simulink model "experiment_toplevel"  (R2016a)
settings: Solver=ode15s  StartTime=0.0  StopTime=20  MaxStep=1e-2  RelTol=1e-4
PreLoadFcn:
  | minitaurParameters
values from neighbouring files (symbols this model uses):
  angular_ctrl_d = 1    [minitaurParameters.m]
  angular_ctrl_i = 1    [minitaurParameters.m]
  angular_ctrl_p = 100    [minitaurParameters.m]
  enc_zero_IA = -1.25*pi    (= -3.92699081699)    [minitaurParameters.m]
  enc_zero_IB = -0.25*pi    (= -0.785398163397)    [minitaurParameters.m]
  enc_zero_IIA = 1.25*pi    (= 3.92699081699)    [minitaurParameters.m]
  enc_zero_IIB = 1.25*pi    (= 3.92699081699)    [minitaurParameters.m]
  enc_zero_IIIA = 0.5*pi    (= 1.57079632679)    [minitaurParameters.m]
  enc_zero_IIIB = 1.5*pi    (= 4.71238898038)    [minitaurParameters.m]
  enc_zero_IVA = -0.25*pi    (= -0.785398163397)    [minitaurParameters.m]
  enc_zero_IVB = 0.5*pi    (= 1.57079632679)    [minitaurParameters.m]
  fore_lag = fore_lag_vals(j)    [experiment1.m]    (also in experiment1_parfor_accelerator.m = 0; minitaurParameters.m = 0.45)
  ground_frame_depth = 0.5    [minitaurParameters.m]
  ground_length = 100    [minitaurParameters.m]
  ground_width = 10    [minitaurParameters.m]
  init_theta_IA = -pi/4    (= -0.785398163397)    [minitaurParameters.m]
  init_theta_IB = pi/4    (= 0.785398163397)    [minitaurParameters.m]
  init_theta_IIA = -pi/4    (= -0.785398163397)    [minitaurParameters.m]
  init_theta_IIB = pi/4    (= 0.785398163397)    [minitaurParameters.m]
  init_theta_IIIA = -pi/4    (= -0.785398163397)    [minitaurParameters.m]
  init_theta_IIIB = pi/4    (= 0.785398163397)    [minitaurParameters.m]
  init_theta_IVA = -pi/4    (= -0.785398163397)    [minitaurParameters.m]
  init_theta_IVB = pi/4    (= 0.785398163397)    [minitaurParameters.m]
  l1 = 100e-3    (= 0.1)    [minitaurParameters.m]
  l2 = 200e-3    (= 0.2)    [minitaurParameters.m]
  leg_joint_radius = 3e-3    (= 0.003)    [minitaurParameters.m]
  lr_sync = 1    [experiment1.m]    (also in experiment1_parfor_accelerator.m; minitaurParameters.m = 0)
  model = 'experiment_toplevel'    [experiment1_parfor_accelerator.m]
  period = period_vals(i)    [experiment1.m]    (also in experiment1_parfor_accelerator.m = 1.5; minitaurParameters.m = 0.33)
  phi_0 = 0.5*asin(l1/l2)    [experiment1.m]    (also in experiment1_parfor_accelerator.m; minitaurParameters.m)
  r_0 = l2    [experiment1.m]    (also in experiment1_parfor_accelerator.m; minitaurParameters.m = 0.2)
  r_x = 0.3*l1    [experiment1.m]    (also in experiment1_parfor_accelerator.m = 0.5*l1; minitaurParameters.m = 0.05)
  r_y = 0.2*l1    [experiment1.m]    (also in experiment1_parfor_accelerator.m = 0.3*l1; minitaurParameters.m = 0.03)
  radial_ctrl_d = 1    [minitaurParameters.m]
  radial_ctrl_i = 1    [minitaurParameters.m]
  radial_ctrl_p = 80    [minitaurParameters.m]
  safety_limit = 10e-3    (= 0.01)    [minitaurParameters.m]
undefined symbols (not defined in the file or in its folder): Axis, Fn, minitaurParams, r_stance, r_swing, stance_frac, X, Y, Z
undefined symbols (not defined in the file): leg_joint_fric_bw, leg_joint_mu_k, leg_joint_mu_s, leg_joint_vel_thresh, motor_kt, motor_kv, motor_r, motor_torque_sat
libraries: sm_lib x453, fl_lib x132, nesl_utility x31, Contact_Forces_Lib x28, simulink x19
(part 2 of 13)

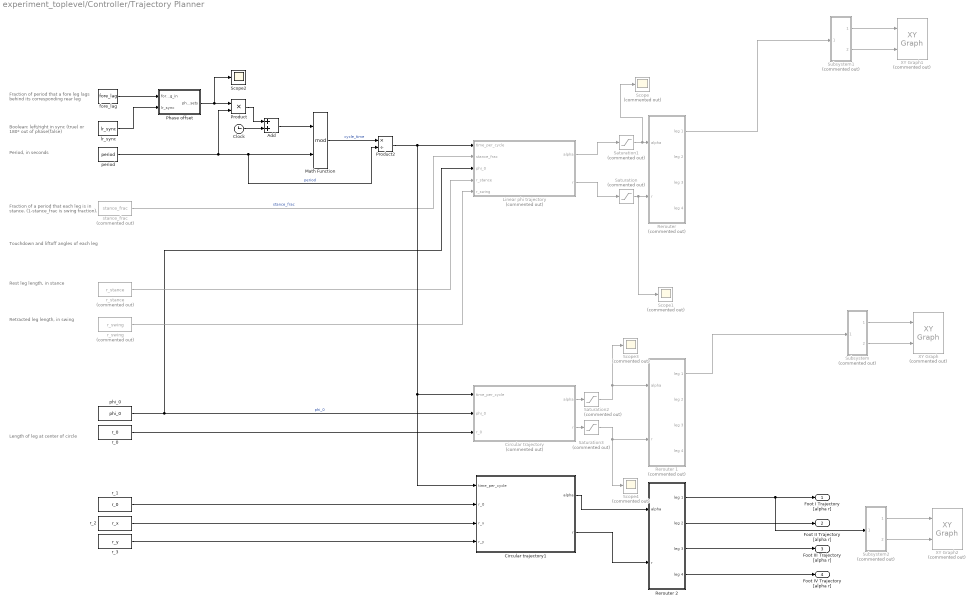
== system experiment_toplevel/Controller/Trajectory Planner ==
  note: Fraction of period that a fore leg
      | lags behind its corresponding rear leg
  note: Period, in seconds
  note: Fraction of a period that each leg is in stance. (1-stance_frac is swing fraction).
  note: Touchdown and liftoff angles of each leg
  note: Boolean: left/right in sync (true) or
      | 180* out of phase(false)
  note: Rest leg length, in stance
  note: Retracted leg length, in swing
  note: Length of leg at center of circle
  Add : Sum
  Circular trajectory : Subsystem  Commented=on
  Circular trajectory1 : Subsystem
  Clock : Clock
  Linear phi trajectory : Subsystem  Commented=on
  Math Function : Math  Operator=mod  SaturateOnIntegerOverflow=on
  Phase offset : Subsystem
  Product : Product
  Product2 : Product  Inputs=*/
  "Rerouter " : Subsystem  Commented=on
  Rerouter 1 : Subsystem  Commented=on
  Rerouter 2 : Subsystem
  Saturation : Saturate  Commented=on  UpperLimit=l2+l1  LowerLimit=l2-l1
  Saturation1 : Saturate  Commented=on  UpperLimit=3*pi/2  LowerLimit=pi/2
  Saturation2 : Saturate  Commented=on  UpperLimit=3*pi/2  LowerLimit=pi/2
  Saturation3 : Saturate  Commented=on  UpperLimit=l2+l1-safety_limit  LowerLimit=l2-l1+safety_limit
  Scope{,1,3..4} (4 alike) : Scope  Commented=on
  Scope2 : Scope
  Subsystem : Subsystem  Commented=on
  Subsystem1 : Subsystem  Commented=on
  Subsystem2 : Subsystem  Commented=on
  XY Graph : simulink/Sinks/XY Graph  Commented=on  xmin=-0.4  xmax=0.4  ymin=-0.5  ymax=0.1  st=-1
  XY Graph1 : simulink/Sinks/XY Graph  Commented=on  xmin=-0.4  xmax=0.4  ymin=-0.5  ymax=0.1  st=-1
  XY Graph2 : simulink/Sinks/XY Graph  Commented=on  xmin=-0.4  xmax=0.4  ymin=-0.5  ymax=0.1  st=-1
  fore_lag : Constant  Value=fore_lag
  lr_sync : Constant  Value=lr_sync  OutDataTypeStr=double
  period : Constant  Value=period  OutDataTypeStr=double
  phi_0 : Constant  Value=phi_0
  r_0 : Constant  Value=r_0
  r_1 : Constant  Value=r_0
  r_2 : Constant  Value=r_x
  r_3 : Constant  Value=r_y
  r_stance : Constant  Commented=on  Value=r_stance
  r_swing : Constant  Commented=on  Value=r_swing
  stance_frac : Constant  Commented=on  Value=stance_frac
  Foot I Trajectory [alpha r] : Outport
  Foot II Trajectory [alpha r] : Outport  Port=2
  Foot III Trajectory [alpha r] : Outport  Port=3
  Foot IV Trajectory [alpha r] : Outport  Port=4
  wires:
  period/1 -> Product/2, Product2/2, Math Function/2  "period"
  Clock/1 -> Add/2
  Add/1 -> Math Function/1
  Product/1 -> Add/1
  Phase offset/1(phase offsets) -> Scope2/1, Product/1
  lr_sync/1 -> Phase offset/2(lr_sync)
  Math Function/1 -> Product2/1  "cycle_time"
  stance_frac/1 -> Linear phi trajectory/2(stance_frac)  "stance_frac"
  phi_0/1 -> Linear phi trajectory/3(phi_0), Circular trajectory/2(phi_0)  "phi_0"
  r_stance/1 -> Linear phi trajectory/4("r_stance ")
  r_swing/1 -> Linear phi trajectory/5(r_swing)
  Product2/1 -> Circular trajectory/1(time_per_cycle), Circular trajectory1/1(time_per_cycle), Linear phi trajectory/1(time_per_cycle)
  r_0/1 -> Circular trajectory/3(r_0)
  Circular trajectory/2(r) -> Saturation3/1
  Subsystem/1(Out1) -> XY Graph/1
  Subsystem/2(Out2) -> XY Graph/2
  Subsystem1/1(Out1) -> XY Graph1/1
  Subsystem1/2(Out2) -> XY Graph1/2
  Saturation/1 -> Scope1/1, "Rerouter "/2(r)
  Saturation1/1 -> Scope/1, "Rerouter "/1(alpha)
  Linear phi trajectory/1(alpha) -> Saturation1/1
  Linear phi trajectory/2(r) -> Saturation/1
  "Rerouter "/1(leg 1) -> Subsystem1/1(In1)
  Circular trajectory/1(alpha) -> Saturation2/1
  Saturation3/1 -> Scope4/1, Rerouter 1/2(r)
  Rerouter 1/1(leg 1) -> Subsystem/1(In1)
  Saturation2/1 -> Scope3/1, Rerouter 1/1(alpha)
  r_1/1 -> Circular trajectory1/2(r_0)
  Circular trajectory1/1(alpha) -> Rerouter 2/1(alpha)
  Circular trajectory1/2(r) -> Rerouter 2/2(r)
  Subsystem2/1(Out1) -> XY Graph2/1
  Subsystem2/2(Out2) -> XY Graph2/2
  Rerouter 2/1(leg 1) -> Foot I Trajectory [alpha r]/1, Subsystem2/1(In1)
  r_2/1 -> Circular trajectory1/3(r_x)
  r_3/1 -> Circular trajectory1/4(r_y)
  Rerouter 2/2(leg 2) -> Foot II Trajectory [alpha r]/1
  Rerouter 2/3(leg 3) -> Foot III Trajectory [alpha r]/1
  Rerouter 2/4(leg 4) -> Foot IV Trajectory [alpha r]/1
  fore_lag/1 -> Phase offset/1(fore_lag_in)

== system experiment_toplevel/Environment/Ground ==
  Ground Track : sm_lib/Body Elements/Solid  InertiaType=CalculateFromGeometry  Mass=1  MassUnits=kg  CenterOfMass=[0 0 0]  CenterOfMassUnits=m  MomentsOfInertia=[1 1 1]  MomentsOfInertiaUnits=kg*m^2  ProductsOfInertia=[0 0 0]  ProductsOfInertiaUnits=kg*m^2  DensityBased=on  Density=1000  DensityUnits=kg/(m^3)  DoExposeReferenceFrame=on  SerializedFrames=<Frames/>  GraphicType=FromGeometry  MarkerShape=Sphere  MarkerSize=10  GraphicVisPropType=SimpleVisualProperties  GraphicDiffuseColor=[0.4 1.0 0.0]  GraphicSpecularColor=[0.5 0.5 0.5 1.0]  GraphicAmbientColor=[0.15 0.15 0.15 1.0]  GraphicEmissiveColor=[0.0 0.0 0.0 1.0]  GraphicShininess=75  GraphicOpacity=1.0  GeometryShape=Brick  RectangleSize=[1 1]  RectangleSizeUnits=m  BrickDimensions=[ground_width ground_length 2*ground_frame_depth]  BrickDimensionUnits=m  CylinderRadius=1  CylinderRadiusUnits=m  CylinderLength=1  CylinderLengthUnits=m  SphereRadius=1  SphereRadiusUnits=m  EllipsoidRadii=[1 1 1]  EllipsoidRadiiUnits=m  ExtrusionCrossSection=[1 1; -1 1; -1 -1; 1 -1]  ExtrusionCrossSectionUnits=m  ExtrusionLength=1  ExtrusionLengthUnits=m  PolygonNumSides=3  PolygonOuterRadius=1  PolygonOuterRadiusUnits=m  ExtGeomFileType=STEP  ExtGeomFileUnits=m  RevolutionCrossSection=[1 1; 1 -1; 2 -1; 2 1]  RevolutionCrossSectionUnits=m  RevolutionExtent=Full  RevolutionAngle=180  RevolutionAngleUnits=deg
  F : PMIOPort  Port=1  Side=Right
  connections:
  F/RConn1 -- Ground Track/RConn1

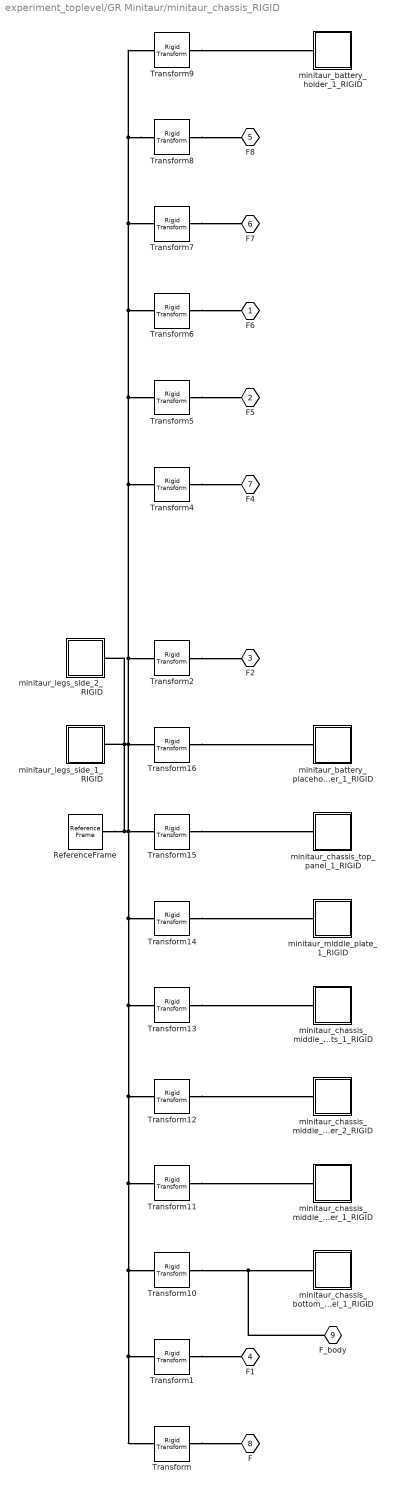
== system experiment_toplevel/GR Minitaur/minitaur_chassis_RIGID ==
  ReferenceFrame : sm_lib/Frames and Transforms/Reference Frame
  Transform : sm_lib/Frames and Transforms/Rigid Transform  TranslationMethod=Cartesian  TranslationLengthUnit=mm  TranslationStandardAxis=+Z  TranslationStandardOffset=0  TranslationCartesianOffset=minitaurParams.RigidTransform(29).translation  TranslationROffset=0  TranslationROffsetUnits=m  TranslationZOffset=0  TranslationZOffsetUnits=m  TranslationThetaOffset=0  TranslationThetaOffsetUnits=deg  RotationMethod=ArbitraryAxis  RotationAngleUnits=rad  RotationStandardAxis=+Z  RotationAngle=minitaurParams.RigidTransform(29).angle  RotationArbitraryAxis=minitaurParams.RigidTransform(29).axis  FollAlignAxisA=+X  BaseAlignAxisA=+Y  FollAlignAxisB=+Y  BaseAlignAxisB=+Z  RotationSequenceAxes=FollowerAxes  RotationSequence=XYX  RotationSequenceAngles=[0 0 0]  RotationSequenceAnglesUnits=deg  RotationMatrix=[1 0 0; 0 1 0; 0 0 1]
  Transform1 : sm_lib/Frames and Transforms/Rigid Transform  TranslationMethod=Cartesian  TranslationLengthUnit=mm  TranslationStandardAxis=+Z  TranslationStandardOffset=0  TranslationCartesianOffset=minitaurParams.RigidTransform(31).translation  TranslationROffset=0  TranslationROffsetUnits=m  TranslationZOffset=0  TranslationZOffsetUnits=m  TranslationThetaOffset=0  TranslationThetaOffsetUnits=deg  RotationMethod=ArbitraryAxis  RotationAngleUnits=rad  RotationStandardAxis=+Z  RotationAngle=minitaurParams.RigidTransform(31).angle  RotationArbitraryAxis=minitaurParams.RigidTransform(31).axis  FollAlignAxisA=+X  BaseAlignAxisA=+Y  FollAlignAxisB=+Y  BaseAlignAxisB=+Z  RotationSequenceAxes=FollowerAxes  RotationSequence=XYX  RotationSequenceAngles=[0 0 0]  RotationSequenceAnglesUnits=deg  RotationMatrix=[1 0 0; 0 1 0; 0 0 1]
  Transform10 : sm_lib/Frames and Transforms/Rigid Transform  TranslationMethod=Cartesian  TranslationLengthUnit=mm  TranslationStandardAxis=+Z  TranslationStandardOffset=0  TranslationCartesianOffset=minitaurParams.RigidTransform(64).translation  TranslationROffset=0  TranslationROffsetUnits=m  TranslationZOffset=0  TranslationZOffsetUnits=m  TranslationThetaOffset=0  TranslationThetaOffsetUnits=deg  RotationMethod=ArbitraryAxis  RotationAngleUnits=rad  RotationStandardAxis=+Z  RotationAngle=minitaurParams.RigidTransform(64).angle  RotationArbitraryAxis=minitaurParams.RigidTransform(64).axis  FollAlignAxisA=+X  BaseAlignAxisA=+Y  FollAlignAxisB=+Y  BaseAlignAxisB=+Z  RotationSequenceAxes=FollowerAxes  RotationSequence=XYX  RotationSequenceAngles=[0 0 0]  RotationSequenceAnglesUnits=deg  RotationMatrix=[1 0 0; 0 1 0; 0 0 1]
  Transform11 : sm_lib/Frames and Transforms/Rigid Transform  TranslationMethod=Cartesian  TranslationLengthUnit=mm  TranslationStandardAxis=+Z  TranslationStandardOffset=0  TranslationCartesianOffset=minitaurParams.RigidTransform(65).translation  TranslationROffset=0  TranslationROffsetUnits=m  TranslationZOffset=0  TranslationZOffsetUnits=m  TranslationThetaOffset=0  TranslationThetaOffsetUnits=deg  RotationMethod=ArbitraryAxis  RotationAngleUnits=rad  RotationStandardAxis=+Z  RotationAngle=minitaurParams.RigidTransform(65).angle  RotationArbitraryAxis=minitaurParams.RigidTransform(65).axis  FollAlignAxisA=+X  BaseAlignAxisA=+Y  FollAlignAxisB=+Y  BaseAlignAxisB=+Z  RotationSequenceAxes=FollowerAxes  RotationSequence=XYX  RotationSequenceAngles=[0 0 0]  RotationSequenceAnglesUnits=deg  RotationMatrix=[1 0 0; 0 1 0; 0 0 1]
  Transform12 : sm_lib/Frames and Transforms/Rigid Transform  TranslationMethod=Cartesian  TranslationLengthUnit=mm  TranslationStandardAxis=+Z  TranslationStandardOffset=0  TranslationCartesianOffset=minitaurParams.RigidTransform(66).translation  TranslationROffset=0  TranslationROffsetUnits=m  TranslationZOffset=0  TranslationZOffsetUnits=m  TranslationThetaOffset=0  TranslationThetaOffsetUnits=deg  RotationMethod=ArbitraryAxis  RotationAngleUnits=rad  RotationStandardAxis=+Z  RotationAngle=minitaurParams.RigidTransform(66).angle  RotationArbitraryAxis=minitaurParams.RigidTransform(66).axis  FollAlignAxisA=+X  BaseAlignAxisA=+Y  FollAlignAxisB=+Y  BaseAlignAxisB=+Z  RotationSequenceAxes=FollowerAxes  RotationSequence=XYX  RotationSequenceAngles=[0 0 0]  RotationSequenceAnglesUnits=deg  RotationMatrix=[1 0 0; 0 1 0; 0 0 1]
  Transform13 : sm_lib/Frames and Transforms/Rigid Transform  TranslationMethod=Cartesian  TranslationLengthUnit=mm  TranslationStandardAxis=+Z  TranslationStandardOffset=0  TranslationCartesianOffset=minitaurParams.RigidTransform(67).translation  TranslationROffset=0  TranslationROffsetUnits=m  TranslationZOffset=0  TranslationZOffsetUnits=m  TranslationThetaOffset=0  TranslationThetaOffsetUnits=deg  RotationMethod=ArbitraryAxis  RotationAngleUnits=rad  RotationStandardAxis=+Z  RotationAngle=minitaurParams.RigidTransform(67).angle  RotationArbitraryAxis=minitaurParams.RigidTransform(67).axis  FollAlignAxisA=+X  BaseAlignAxisA=+Y  FollAlignAxisB=+Y  BaseAlignAxisB=+Z  RotationSequenceAxes=FollowerAxes  RotationSequence=XYX  RotationSequenceAngles=[0 0 0]  RotationSequenceAnglesUnits=deg  RotationMatrix=[1 0 0; 0 1 0; 0 0 1]
  Transform14 : sm_lib/Frames and Transforms/Rigid Transform  TranslationMethod=Cartesian  TranslationLengthUnit=mm  TranslationStandardAxis=+Z  TranslationStandardOffset=0  TranslationCartesianOffset=minitaurParams.RigidTransform(68).translation  TranslationROffset=0  TranslationROffsetUnits=m  TranslationZOffset=0  TranslationZOffsetUnits=m  TranslationThetaOffset=0  TranslationThetaOffsetUnits=deg  RotationMethod=ArbitraryAxis  RotationAngleUnits=rad  RotationStandardAxis=+Z  RotationAngle=minitaurParams.RigidTransform(68).angle  RotationArbitraryAxis=minitaurParams.RigidTransform(68).axis  FollAlignAxisA=+X  BaseAlignAxisA=+Y  FollAlignAxisB=+Y  BaseAlignAxisB=+Z  RotationSequenceAxes=FollowerAxes  RotationSequence=XYX  RotationSequenceAngles=[0 0 0]  RotationSequenceAnglesUnits=deg  RotationMatrix=[1 0 0; 0 1 0; 0 0 1]
  Transform15 : sm_lib/Frames and Transforms/Rigid Transform  TranslationMethod=Cartesian  TranslationLengthUnit=mm  TranslationStandardAxis=+Z  TranslationStandardOffset=0  TranslationCartesianOffset=minitaurParams.RigidTransform(69).translation  TranslationROffset=0  TranslationROffsetUnits=m  TranslationZOffset=0  TranslationZOffsetUnits=m  TranslationThetaOffset=0  TranslationThetaOffsetUnits=deg  RotationMethod=ArbitraryAxis  RotationAngleUnits=rad  RotationStandardAxis=+Z  RotationAngle=minitaurParams.RigidTransform(69).angle  RotationArbitraryAxis=minitaurParams.RigidTransform(69).axis  FollAlignAxisA=+X  BaseAlignAxisA=+Y  FollAlignAxisB=+Y  BaseAlignAxisB=+Z  RotationSequenceAxes=FollowerAxes  RotationSequence=XYX  RotationSequenceAngles=[0 0 0]  RotationSequenceAnglesUnits=deg  RotationMatrix=[1 0 0; 0 1 0; 0 0 1]
  Transform16 : sm_lib/Frames and Transforms/Rigid Transform  TranslationMethod=Cartesian  TranslationLengthUnit=mm  TranslationStandardAxis=+Z  TranslationStandardOffset=0  TranslationCartesianOffset=minitaurParams.RigidTransform(86).translation  TranslationROffset=0  TranslationROffsetUnits=m  TranslationZOffset=0  TranslationZOffsetUnits=m  TranslationThetaOffset=0  TranslationThetaOffsetUnits=deg  RotationMethod=ArbitraryAxis  RotationAngleUnits=rad  RotationStandardAxis=+Z  RotationAngle=minitaurParams.RigidTransform(86).angle  RotationArbitraryAxis=minitaurParams.RigidTransform(86).axis  FollAlignAxisA=+X  BaseAlignAxisA=+Y  FollAlignAxisB=+Y  BaseAlignAxisB=+Z  RotationSequenceAxes=FollowerAxes  RotationSequence=XYX  RotationSequenceAngles=[0 0 0]  RotationSequenceAnglesUnits=deg  RotationMatrix=[1 0 0; 0 1 0; 0 0 1]
  Transform2 : sm_lib/Frames and Transforms/Rigid Transform  TranslationMethod=Cartesian  TranslationLengthUnit=mm  TranslationStandardAxis=+Z  TranslationStandardOffset=0  TranslationCartesianOffset=minitaurParams.RigidTransform(33).translation  TranslationROffset=0  TranslationROffsetUnits=m  TranslationZOffset=0  TranslationZOffsetUnits=m  TranslationThetaOffset=0  TranslationThetaOffsetUnits=deg  RotationMethod=ArbitraryAxis  RotationAngleUnits=rad  RotationStandardAxis=+Z  RotationAngle=minitaurParams.RigidTransform(33).angle  RotationArbitraryAxis=minitaurParams.RigidTransform(33).axis  FollAlignAxisA=+X  BaseAlignAxisA=+Y  FollAlignAxisB=+Y  BaseAlignAxisB=+Z  RotationSequenceAxes=FollowerAxes  RotationSequence=XYX  RotationSequenceAngles=[0 0 0]  RotationSequenceAnglesUnits=deg  RotationMatrix=[1 0 0; 0 1 0; 0 0 1]
  Transform4 : sm_lib/Frames and Transforms/Rigid Transform  TranslationMethod=Cartesian  TranslationLengthUnit=mm  TranslationStandardAxis=+Z  TranslationStandardOffset=0  TranslationCartesianOffset=minitaurParams.RigidTransform(37).translation  TranslationROffset=0  TranslationROffsetUnits=m  TranslationZOffset=0  TranslationZOffsetUnits=m  TranslationThetaOffset=0  TranslationThetaOffsetUnits=deg  RotationMethod=ArbitraryAxis  RotationAngleUnits=rad  RotationStandardAxis=+Z  RotationAngle=minitaurParams.RigidTransform(37).angle  RotationArbitraryAxis=minitaurParams.RigidTransform(37).axis  FollAlignAxisA=+X  BaseAlignAxisA=+Y  FollAlignAxisB=+Y  BaseAlignAxisB=+Z  RotationSequenceAxes=FollowerAxes  RotationSequence=XYX  RotationSequenceAngles=[0 0 0]  RotationSequenceAnglesUnits=deg  RotationMatrix=[1 0 0; 0 1 0; 0 0 1]
  Transform5 : sm_lib/Frames and Transforms/Rigid Transform  TranslationMethod=Cartesian  TranslationLengthUnit=mm  TranslationStandardAxis=+Z  TranslationStandardOffset=0  TranslationCartesianOffset=minitaurParams.RigidTransform(39).translation  TranslationROffset=0  TranslationROffsetUnits=m  TranslationZOffset=0  TranslationZOffsetUnits=m  TranslationThetaOffset=0  TranslationThetaOffsetUnits=deg  RotationMethod=ArbitraryAxis  RotationAngleUnits=rad  RotationStandardAxis=+Z  RotationAngle=minitaurParams.RigidTransform(39).angle  RotationArbitraryAxis=minitaurParams.RigidTransform(39).axis  FollAlignAxisA=+X  BaseAlignAxisA=+Y  FollAlignAxisB=+Y  BaseAlignAxisB=+Z  RotationSequenceAxes=FollowerAxes  RotationSequence=XYX  RotationSequenceAngles=[0 0 0]  RotationSequenceAnglesUnits=deg  RotationMatrix=[1 0 0; 0 1 0; 0 0 1]
  Transform6 : sm_lib/Frames and Transforms/Rigid Transform  TranslationMethod=Cartesian  TranslationLengthUnit=mm  TranslationStandardAxis=+Z  TranslationStandardOffset=0  TranslationCartesianOffset=minitaurParams.RigidTransform(41).translation  TranslationROffset=0  TranslationROffsetUnits=m  TranslationZOffset=0  TranslationZOffsetUnits=m  TranslationThetaOffset=0  TranslationThetaOffsetUnits=deg  RotationMethod=ArbitraryAxis  RotationAngleUnits=rad  RotationStandardAxis=+Z  RotationAngle=minitaurParams.RigidTransform(41).angle  RotationArbitraryAxis=minitaurParams.RigidTransform(41).axis  FollAlignAxisA=+X  BaseAlignAxisA=+Y  FollAlignAxisB=+Y  BaseAlignAxisB=+Z  RotationSequenceAxes=FollowerAxes  RotationSequence=XYX  RotationSequenceAngles=[0 0 0]  RotationSequenceAnglesUnits=deg  RotationMatrix=[1 0 0; 0 1 0; 0 0 1]
  Transform7 : sm_lib/Frames and Transforms/Rigid Transform  TranslationMethod=Cartesian  TranslationLengthUnit=mm  TranslationStandardAxis=+Z  TranslationStandardOffset=0  TranslationCartesianOffset=minitaurParams.RigidTransform(55).translation  TranslationROffset=0  TranslationROffsetUnits=m  TranslationZOffset=0  TranslationZOffsetUnits=m  TranslationThetaOffset=0  TranslationThetaOffsetUnits=deg  RotationMethod=ArbitraryAxis  RotationAngleUnits=rad  RotationStandardAxis=+Z  RotationAngle=minitaurParams.RigidTransform(55).angle  RotationArbitraryAxis=minitaurParams.RigidTransform(55).axis  FollAlignAxisA=+X  BaseAlignAxisA=+Y  FollAlignAxisB=+Y  BaseAlignAxisB=+Z  RotationSequenceAxes=FollowerAxes  RotationSequence=XYX  RotationSequenceAngles=[0 0 0]  RotationSequenceAnglesUnits=deg  RotationMatrix=[1 0 0; 0 1 0; 0 0 1]
  Transform8 : sm_lib/Frames and Transforms/Rigid Transform  TranslationMethod=Cartesian  TranslationLengthUnit=mm  TranslationStandardAxis=+Z  TranslationStandardOffset=0  TranslationCartesianOffset=minitaurParams.RigidTransform(61).translation  TranslationROffset=0  TranslationROffsetUnits=m  TranslationZOffset=0  TranslationZOffsetUnits=m  TranslationThetaOffset=0  TranslationThetaOffsetUnits=deg  RotationMethod=ArbitraryAxis  RotationAngleUnits=rad  RotationStandardAxis=+Z  RotationAngle=minitaurParams.RigidTransform(61).angle  RotationArbitraryAxis=minitaurParams.RigidTransform(61).axis  FollAlignAxisA=+X  BaseAlignAxisA=+Y  FollAlignAxisB=+Y  BaseAlignAxisB=+Z  RotationSequenceAxes=FollowerAxes  RotationSequence=XYX  RotationSequenceAngles=[0 0 0]  RotationSequenceAnglesUnits=deg  RotationMatrix=[1 0 0; 0 1 0; 0 0 1]
  Transform9 : sm_lib/Frames and Transforms/Rigid Transform  TranslationMethod=Cartesian  TranslationLengthUnit=mm  TranslationStandardAxis=+Z  TranslationStandardOffset=0  TranslationCartesianOffset=minitaurParams.RigidTransform(63).translation  TranslationROffset=0  TranslationROffsetUnits=m  TranslationZOffset=0  TranslationZOffsetUnits=m  TranslationThetaOffset=0  TranslationThetaOffsetUnits=deg  RotationMethod=ArbitraryAxis  RotationAngleUnits=rad  RotationStandardAxis=+Z  RotationAngle=minitaurParams.RigidTransform(63).angle  RotationArbitraryAxis=minitaurParams.RigidTransform(63).axis  FollAlignAxisA=+X  BaseAlignAxisA=+Y  FollAlignAxisB=+Y  BaseAlignAxisB=+Z  RotationSequenceAxes=FollowerAxes  RotationSequence=XYX  RotationSequenceAngles=[0 0 0]  RotationSequenceAnglesUnits=deg  RotationMatrix=[1 0 0; 0 1 0; 0 0 1]
  minitaur_battery_holder_1_RIGID : Subsystem
  minitaur_battery_placeholder_1_RIGID : Subsystem
  minitaur_chassis_bottom_panel_1_RIGID : Subsystem
  minitaur_chassis_middle_plate_plastic_cover_1_RIGID : Subsystem
  minitaur_chassis_middle_plate_plastic_cover_2_RIGID : Subsystem
  minitaur_chassis_middle_plate_plastic_cover_cutouts_1_RIGID : Subsystem
  minitaur_chassis_top_panel_1_RIGID : Subsystem
  minitaur_legs_side_1_RIGID : Subsystem
  minitaur_legs_side_2_RIGID : Subsystem
  minitaur_middle_plate_1_RIGID : Subsystem
  F6 : PMIOPort  Port=1  Side=Left
  F5 : PMIOPort  Port=2  Side=Left
  F2 : PMIOPort  Port=3  Side=Left
  F1 : PMIOPort  Port=4  Side=Left
  F8 : PMIOPort  Port=5  Side=Left
  F7 : PMIOPort  Port=6  Side=Left
  F4 : PMIOPort  Port=7  Side=Left
  F : PMIOPort  Port=8  Side=Left
  F_body : PMIOPort  Port=9  Side=Right
  connections:
  Transform8/LConn1 -- Transform9/LConn1 -- Transform/LConn1 -- Transform1/LConn1 -- Transform10/LConn1 -- Transform11/LConn1 -- Transform12/LConn1 -- Transform13/LConn1 -- Transform14/LConn1 -- ReferenceFrame/RConn1 -- minitaur_legs_side_1_RIGID/RConn1 -- minitaur_legs_side_2_RIGID/RConn1 -- Transform15/LConn1 -- Transform16/LConn1 -- Transform2/LConn1 -- Transform4/LConn1 -- Transform5/LConn1 -- Transform6/LConn1 -- Transform7/LConn1
  Transform/RConn1 -- F/RConn1
  Transform9/RConn1 -- minitaur_battery_holder_1_RIGID/LConn1
  Transform10/RConn1 -- F_body/RConn1 -- minitaur_chassis_bottom_panel_1_RIGID/LConn1
  Transform11/RConn1 -- minitaur_chassis_middle_plate_plastic_cover_1_RIGID/LConn1
  Transform12/RConn1 -- minitaur_chassis_middle_plate_plastic_cover_2_RIGID/LConn1
  Transform13/RConn1 -- minitaur_chassis_middle_plate_plastic_cover_cutouts_1_RIGID/LConn1
  Transform14/RConn1 -- minitaur_middle_plate_1_RIGID/LConn1
  Transform15/RConn1 -- minitaur_chassis_top_panel_1_RIGID/LConn1
  Transform16/RConn1 -- minitaur_battery_placeholder_1_RIGID/LConn1
  Transform1/RConn1 -- F1/RConn1
  Transform2/RConn1 -- F2/RConn1
  Transform4/RConn1 -- F4/RConn1
  Transform5/RConn1 -- F5/RConn1
  Transform6/RConn1 -- F6/RConn1
  Transform7/RConn1 -- F7/RConn1
  Transform8/RConn1 -- F8/RConn1

== system experiment_toplevel/GR Minitaur/minitaur_leg_linkages_I ==
  Joint Friction Model : Subsystem  Variant=on  OverrideUsingVariant=stick-slip  mask(Joint Friction Model){modelVariant=Stick-Slip Friction, leg_joint_radius=leg_joint_radius, linear_region_thresh=leg_joint_vel_thresh, mu_k=leg_joint_mu_k, mu_s=leg_joint_mu_s, fric_bandwidth=leg_joint_fric_bw, mu_brk=0, fric_visc_coeff=0, trans_coeff=0}
      mask prompts: modelVariant "Friction Model"; leg_joint_radius "Leg Joint Effective Radius [m]"; linear_region_thresh "Linear Region Velocity Threshold [m/s]"; mu_k "Kinetic Friction Coefficient []"; mu_s "Static Friction Coefficient []"; fric_bandwidth "Friction Model Bandwidth [Hz]"; mu_brk "Breakaway Friction Coefficient []"; fric_visc_coeff "Viscous Friction Coefficient [N*s/m]"; trans_coeff "Transition Approximation Coefficient [s/m]"
      mask help: Models rotational friction present in passive joints. Two options available: stick-slip, and an advanced model that includes viscous and Stribeck friction. Note that in all models, friction is calculated as translational force couple, which is then converted to a friction torque (multiplied by effective joint diameter).
      mask TypeOptions modelVariant: Full Friction | Stick-Slip Friction
      mask Callback modelVariant:
      | currVariant = get_param(gcb,'modelVariant')
      | 
      | switch currVariant
      |     case 'Stick-Slip Friction'
      |         set_param(gcb,'OverrideUsingVariant','stick-slip')
      |         set_param(gcb,'MaskVisibilities',{'on';'on';'on';'on';'on';'on';'off';'off';'off'})
      |     case 'Full Friction'
      |         set_param(gcb,'OverrideUsingVariant','full')
      |         set_param(gcb,'MaskVisibilities',{'on';'on';'on';'on';'off';'off';'on';'on';'on'})
      | 
      | end
  Joint Friction Model1 : Subsystem  Variant=on  OverrideUsingVariant=stick-slip  mask(Joint Friction Model){modelVariant=Stick-Slip Friction, leg_joint_radius=leg_joint_radius, linear_region_thresh=leg_joint_vel_thresh, mu_k=leg_joint_mu_k, mu_s=leg_joint_mu_s, fric_bandwidth=leg_joint_fric_bw, mu_brk=0, fric_visc_coeff=0, trans_coeff=0}
      mask prompts: modelVariant "Friction Model"; leg_joint_radius "Leg Joint Effective Radius [m]"; linear_region_thresh "Linear Region Velocity Threshold [m/s]"; mu_k "Kinetic Friction Coefficient []"; mu_s "Static Friction Coefficient []"; fric_bandwidth "Friction Model Bandwidth [Hz]"; mu_brk "Breakaway Friction Coefficient []"; fric_visc_coeff "Viscous Friction Coefficient [N*s/m]"; trans_coeff "Transition Approximation Coefficient [s/m]"
      mask help: Models rotational friction present in passive joints. Two options available: stick-slip, and an advanced model that includes viscous and Stribeck friction. Note that in all models, friction is calculated as translational force couple, which is then converted to a friction torque (multiplied by effective joint diameter).
      mask TypeOptions modelVariant: Full Friction | Stick-Slip Friction
      mask Callback modelVariant:
      | currVariant = get_param(gcb,'modelVariant')
      | 
      | switch currVariant
      |     case 'Stick-Slip Friction'
      |         set_param(gcb,'OverrideUsingVariant','stick-slip')
      |         set_param(gcb,'MaskVisibilities',{'on';'on';'on';'on';'on';'on';'off';'off';'off'})
      |     case 'Full Friction'
      |         set_param(gcb,'OverrideUsingVariant','full')
      |         set_param(gcb,'MaskVisibilities',{'on';'on';'on';'on';'off';'off';'on';'on';'on'})
      | 
      | end
  Joint Friction Model2 : Subsystem  Variant=on  OverrideUsingVariant=stick-slip  mask(Joint Friction Model){modelVariant=Stick-Slip Friction, leg_joint_radius=leg_joint_radius, linear_region_thresh=leg_joint_vel_thresh, mu_k=leg_joint_mu_k, mu_s=leg_joint_mu_s, fric_bandwidth=leg_joint_fric_bw, mu_brk=0, fric_visc_coeff=0, trans_coeff=0}
      mask prompts: modelVariant "Friction Model"; leg_joint_radius "Leg Joint Effective Radius [m]"; linear_region_thresh "Linear Region Velocity Threshold [m/s]"; mu_k "Kinetic Friction Coefficient []"; mu_s "Static Friction Coefficient []"; fric_bandwidth "Friction Model Bandwidth [Hz]"; mu_brk "Breakaway Friction Coefficient []"; fric_visc_coeff "Viscous Friction Coefficient [N*s/m]"; trans_coeff "Transition Approximation Coefficient [s/m]"
      mask help: Models rotational friction present in passive joints. Two options available: stick-slip, and an advanced model that includes viscous and Stribeck friction. Note that in all models, friction is calculated as translational force couple, which is then converted to a friction torque (multiplied by effective joint diameter).
      mask TypeOptions modelVariant: Full Friction | Stick-Slip Friction
      mask Callback modelVariant:
      | currVariant = get_param(gcb,'modelVariant')
      | 
      | switch currVariant
      |     case 'Stick-Slip Friction'
      |         set_param(gcb,'OverrideUsingVariant','stick-slip')
      |         set_param(gcb,'MaskVisibilities',{'on';'on';'on';'on';'on';'on';'off';'off';'off'})
      |     case 'Full Friction'
      |         set_param(gcb,'OverrideUsingVariant','full')
      |         set_param(gcb,'MaskVisibilities',{'on';'on';'on';'on';'off';'off';'on';'on';'on'})
      | 
      | end
  ReferenceFrame : sm_lib/Frames and Transforms/Reference Frame
  Revolute1 : sm_lib/Joints/Revolute Joint  SenseConstraintForce=off  SenseConstraintForceX=off  SenseConstraintForceY=off  SenseConstraintForceZ=off  SenseConstraintTorque=off  SenseConstraintTorqueX=off  SenseConstraintTorqueY=off  SenseConstraintTorqueZ=off  SenseTotalForce=on  SenseTotalForceX=off  SenseTotalForceY=off  SenseTotalForceZ=off  SenseTotalTorque=off  SenseTotalTorqueX=off  SenseTotalTorqueY=off  SenseTotalTorqueZ=off  CompositeWrenchDir=FollowerOnBase  CompositeWrenchFrame=BaseFrame  EquilibriumPosition=0  EquilibriumPositionUnits=rad  SpringStiffness=0  SpringStiffnessUnits=m*N/rad  DampingCoefficient=0  DampingCoefficientUnits=m*s*N/rad  TorqueActuationMode=InputTorque  MotionActuationMode=ComputedMotion  SensePosition=off  SenseVelocity=on  SenseAcceleration=off  SenseTorqueForce=off  PositionTargetSpecify=on  PositionTargetPriority=Low  PositionTargetValue=init_toe_joint_r  PositionTargetValueUnits=rad  VelocityTargetSpecify=off  VelocityTargetPriority=High  VelocityTargetValue=0  VelocityTargetValueUnits=deg/s
  Revolute2 : sm_lib/Joints/Revolute Joint  SenseConstraintForce=off  SenseConstraintForceX=off  SenseConstraintForceY=off  SenseConstraintForceZ=off  SenseConstraintTorque=off  SenseConstraintTorqueX=off  SenseConstraintTorqueY=off  SenseConstraintTorqueZ=off  SenseTotalForce=on  SenseTotalForceX=off  SenseTotalForceY=off  SenseTotalForceZ=off  SenseTotalTorque=off  SenseTotalTorqueX=off  SenseTotalTorqueY=off  SenseTotalTorqueZ=off  CompositeWrenchDir=FollowerOnBase  CompositeWrenchFrame=BaseFrame  EquilibriumPosition=0  EquilibriumPositionUnits=rad  SpringStiffness=0  SpringStiffnessUnits=m*N/rad  DampingCoefficient=0  DampingCoefficientUnits=m*s*N/rad  TorqueActuationMode=InputTorque  MotionActuationMode=ComputedMotion  SensePosition=off  SenseVelocity=on  SenseAcceleration=off  SenseTorqueForce=off  PositionTargetSpecify=off  PositionTargetPriority=Low  PositionTargetValue=minitaurParams.RevoluteJoint(3).Rz.Pos  PositionTargetValueUnits=deg  VelocityTargetSpecify=off  VelocityTargetPriority=High  VelocityTargetValue=0  VelocityTargetValueUnits=deg/s
  Revolute3 : sm_lib/Joints/Revolute Joint  SenseConstraintForce=off  SenseConstraintForceX=off  SenseConstraintForceY=off  SenseConstraintForceZ=off  SenseConstraintTorque=off  SenseConstraintTorqueX=off  SenseConstraintTorqueY=off  SenseConstraintTorqueZ=off  SenseTotalForce=on  SenseTotalForceX=off  SenseTotalForceY=off  SenseTotalForceZ=off  SenseTotalTorque=off  SenseTotalTorqueX=off  SenseTotalTorqueY=off  SenseTotalTorqueZ=off  CompositeWrenchDir=FollowerOnBase  CompositeWrenchFrame=BaseFrame  EquilibriumPosition=0  EquilibriumPositionUnits=rad  SpringStiffness=0  SpringStiffnessUnits=m*N/rad  DampingCoefficient=0  DampingCoefficientUnits=m*s*N/rad  TorqueActuationMode=InputTorque  MotionActuationMode=ComputedMotion  SensePosition=off  SenseVelocity=on  SenseAcceleration=off  SenseTorqueForce=off  PositionTargetSpecify=off  PositionTargetPriority=Low  PositionTargetValue=minitaurParams.RevoluteJoint(3).Rz.Pos  PositionTargetValueUnits=deg  VelocityTargetSpecify=off  VelocityTargetPriority=High  VelocityTargetValue=0  VelocityTargetValueUnits=deg/s
  Transform : sm_lib/Frames and Transforms/Rigid Transform  TranslationMethod=Cartesian  TranslationLengthUnit=mm  TranslationStandardAxis=+Z  TranslationStandardOffset=0  TranslationCartesianOffset=minitaurParams.RigidTransform(16).translation  TranslationROffset=0  TranslationROffsetUnits=m  TranslationZOffset=0  TranslationZOffsetUnits=m  TranslationThetaOffset=0  TranslationThetaOffsetUnits=deg  RotationMethod=ArbitraryAxis  RotationAngleUnits=rad  RotationStandardAxis=+Z  RotationAngle=minitaurParams.RigidTransform(16).angle  RotationArbitraryAxis=minitaurParams.RigidTransform(16).axis  FollAlignAxisA=+X  BaseAlignAxisA=+Y  FollAlignAxisB=+Y  BaseAlignAxisB=+Z  RotationSequenceAxes=FollowerAxes  RotationSequence=XYX  RotationSequenceAngles=[0 0 0]  RotationSequenceAnglesUnits=deg  RotationMatrix=[1 0 0; 0 1 0; 0 0 1]
  minitaur_leg_joint_placeholder_sim_1_RIGID : Subsystem
  minitaur_leg_joint_placeholder_sim_2_RIGID : Subsystem
  minitaur_leg_joint_placeholder_sim_3_RIGID : Subsystem
  minitaur_leg_lower_link_1_RIGID : Subsystem
  minitaur_leg_lower_link_toe_1_RIGID : Subsystem
  minitaur_leg_upper_link_2_RIGID : Subsystem
  minitaur_leg_upper_link_3_RIGID : Subsystem
  x2517T32_2_RIGID : Subsystem
  F1 : PMIOPort  Port=1  Side=Left
  F : PMIOPort  Port=2  Side=Left
  F_contact : PMIOPort  Port=3  Side=Right
  connections:
  Revolute3/LConn1 -- minitaur_leg_upper_link_3_RIGID/RConn1
  Revolute3/RConn1 -- minitaur_leg_lower_link_1_RIGID/LConn2
  ReferenceFrame/RConn1 -- Transform/LConn1
  Transform/RConn1 -- minitaur_leg_upper_link_2_RIGID/LConn1
  minitaur_leg_upper_link_2_RIGID/LConn2 -- F/RConn1
  minitaur_leg_upper_link_3_RIGID/LConn1 -- F1/RConn1
  Revolute1/LConn1 -- minitaur_leg_lower_link_toe_1_RIGID/RConn2
  Revolute1/RConn1 -- minitaur_leg_lower_link_1_RIGID/LConn1
  minitaur_leg_joint_placeholder_sim_2_RIGID/LConn1 -- minitaur_leg_lower_link_toe_1_RIGID/LConn2
  Revolute2/LConn1 -- minitaur_leg_lower_link_toe_1_RIGID/RConn1
  Revolute2/RConn1 -- minitaur_leg_upper_link_2_RIGID/LConn3
  minitaur_leg_lower_link_toe_1_RIGID/LConn1 -- x2517T32_2_RIGID/LConn1
  minitaur_leg_joint_placeholder_sim_1_RIGID/LConn1 -- minitaur_leg_upper_link_3_RIGID/LConn2
  minitaur_leg_joint_placeholder_sim_3_RIGID/LConn1 -- minitaur_leg_upper_link_2_RIGID/LConn4
  Revolute2/LConn2 -- Joint Friction Model/RConn1
  F_contact/RConn1 -- x2517T32_2_RIGID/RConn1
  Revolute2/RConn2 -- Joint Friction Model/LConn1
  Revolute2/RConn3 -- Joint Friction Model/LConn2
  Revolute1/RConn2 -- Joint Friction Model1/LConn1
  Revolute1/LConn2 -- Joint Friction Model1/RConn1
  Revolute1/RConn3 -- Joint Friction Model1/LConn2
  Revolute3/LConn2 -- Joint Friction Model2/RConn1
  Revolute3/RConn3 -- Joint Friction Model2/LConn2
  Revolute3/RConn2 -- Joint Friction Model2/LConn1

== system experiment_toplevel/GR Minitaur/minitaur_leg_linkages_II ==
  Joint Friction Model : Subsystem  Variant=on  OverrideUsingVariant=stick-slip  mask(Joint Friction Model){modelVariant=Stick-Slip Friction, leg_joint_radius=leg_joint_radius, linear_region_thresh=leg_joint_vel_thresh, mu_k=leg_joint_mu_k, mu_s=leg_joint_mu_s, fric_bandwidth=leg_joint_fric_bw, mu_brk=0, fric_visc_coeff=0, trans_coeff=0}
      mask prompts: modelVariant "Friction Model"; leg_joint_radius "Leg Joint Effective Radius [m]"; linear_region_thresh "Linear Region Velocity Threshold [m/s]"; mu_k "Kinetic Friction Coefficient []"; mu_s "Static Friction Coefficient []"; fric_bandwidth "Friction Model Bandwidth [Hz]"; mu_brk "Breakaway Friction Coefficient []"; fric_visc_coeff "Viscous Friction Coefficient [N*s/m]"; trans_coeff "Transition Approximation Coefficient [s/m]"
      mask help: Models rotational friction present in passive joints. Two options available: stick-slip, and an advanced model that includes viscous and Stribeck friction. Note that in all models, friction is calculated as translational force couple, which is then converted to a friction torque (multiplied by effective joint diameter).
      mask TypeOptions modelVariant: Full Friction | Stick-Slip Friction
      mask Callback modelVariant:
      | currVariant = get_param(gcb,'modelVariant')
      | 
      | switch currVariant
      |     case 'Stick-Slip Friction'
      |         set_param(gcb,'OverrideUsingVariant','stick-slip')
      |         set_param(gcb,'MaskVisibilities',{'on';'on';'on';'on';'on';'on';'off';'off';'off'})
      |     case 'Full Friction'
      |         set_param(gcb,'OverrideUsingVariant','full')
      |         set_param(gcb,'MaskVisibilities',{'on';'on';'on';'on';'off';'off';'on';'on';'on'})
      | 
      | end
  Joint Friction Model1 : Subsystem  Variant=on  OverrideUsingVariant=stick-slip  mask(Joint Friction Model){modelVariant=Stick-Slip Friction, leg_joint_radius=leg_joint_radius, linear_region_thresh=leg_joint_vel_thresh, mu_k=leg_joint_mu_k, mu_s=leg_joint_mu_s, fric_bandwidth=leg_joint_fric_bw, mu_brk=0, fric_visc_coeff=0, trans_coeff=0}
      mask prompts: modelVariant "Friction Model"; leg_joint_radius "Leg Joint Effective Radius [m]"; linear_region_thresh "Linear Region Velocity Threshold [m/s]"; mu_k "Kinetic Friction Coefficient []"; mu_s "Static Friction Coefficient []"; fric_bandwidth "Friction Model Bandwidth [Hz]"; mu_brk "Breakaway Friction Coefficient []"; fric_visc_coeff "Viscous Friction Coefficient [N*s/m]"; trans_coeff "Transition Approximation Coefficient [s/m]"
      mask help: Models rotational friction present in passive joints. Two options available: stick-slip, and an advanced model that includes viscous and Stribeck friction. Note that in all models, friction is calculated as translational force couple, which is then converted to a friction torque (multiplied by effective joint diameter).
      mask TypeOptions modelVariant: Full Friction | Stick-Slip Friction
      mask Callback modelVariant:
      | currVariant = get_param(gcb,'modelVariant')
      | 
      | switch currVariant
      |     case 'Stick-Slip Friction'
      |         set_param(gcb,'OverrideUsingVariant','stick-slip')
      |         set_param(gcb,'MaskVisibilities',{'on';'on';'on';'on';'on';'on';'off';'off';'off'})
      |     case 'Full Friction'
      |         set_param(gcb,'OverrideUsingVariant','full')
      |         set_param(gcb,'MaskVisibilities',{'on';'on';'on';'on';'off';'off';'on';'on';'on'})
      | 
      | end
  Joint Friction Model2 : Subsystem  Variant=on  OverrideUsingVariant=stick-slip  mask(Joint Friction Model){modelVariant=Stick-Slip Friction, leg_joint_radius=leg_joint_radius, linear_region_thresh=leg_joint_vel_thresh, mu_k=leg_joint_mu_k, mu_s=leg_joint_mu_s, fric_bandwidth=leg_joint_fric_bw, mu_brk=0, fric_visc_coeff=0, trans_coeff=0}
      mask prompts: modelVariant "Friction Model"; leg_joint_radius "Leg Joint Effective Radius [m]"; linear_region_thresh "Linear Region Velocity Threshold [m/s]"; mu_k "Kinetic Friction Coefficient []"; mu_s "Static Friction Coefficient []"; fric_bandwidth "Friction Model Bandwidth [Hz]"; mu_brk "Breakaway Friction Coefficient []"; fric_visc_coeff "Viscous Friction Coefficient [N*s/m]"; trans_coeff "Transition Approximation Coefficient [s/m]"
      mask help: Models rotational friction present in passive joints. Two options available: stick-slip, and an advanced model that includes viscous and Stribeck friction. Note that in all models, friction is calculated as translational force couple, which is then converted to a friction torque (multiplied by effective joint diameter).
      mask TypeOptions modelVariant: Full Friction | Stick-Slip Friction
      mask Callback modelVariant:
      | currVariant = get_param(gcb,'modelVariant')
      | 
      | switch currVariant
      |     case 'Stick-Slip Friction'
      |         set_param(gcb,'OverrideUsingVariant','stick-slip')
      |         set_param(gcb,'MaskVisibilities',{'on';'on';'on';'on';'on';'on';'off';'off';'off'})
      |     case 'Full Friction'
      |         set_param(gcb,'OverrideUsingVariant','full')
      |         set_param(gcb,'MaskVisibilities',{'on';'on';'on';'on';'off';'off';'on';'on';'on'})
      | 
      | end
  ReferenceFrame : sm_lib/Frames and Transforms/Reference Frame
  Revolute1 : sm_lib/Joints/Revolute Joint  SenseConstraintForce=off  SenseConstraintForceX=off  SenseConstraintForceY=off  SenseConstraintForceZ=off  SenseConstraintTorque=off  SenseConstraintTorqueX=off  SenseConstraintTorqueY=off  SenseConstraintTorqueZ=off  SenseTotalForce=on  SenseTotalForceX=off  SenseTotalForceY=off  SenseTotalForceZ=off  SenseTotalTorque=off  SenseTotalTorqueX=off  SenseTotalTorqueY=off  SenseTotalTorqueZ=off  CompositeWrenchDir=FollowerOnBase  CompositeWrenchFrame=BaseFrame  EquilibriumPosition=0  EquilibriumPositionUnits=rad  SpringStiffness=0  SpringStiffnessUnits=m*N/rad  DampingCoefficient=0  DampingCoefficientUnits=m*s*N/rad  TorqueActuationMode=InputTorque  MotionActuationMode=ComputedMotion  SensePosition=off  SenseVelocity=on  SenseAcceleration=off  SenseTorqueForce=off  PositionTargetSpecify=on  PositionTargetPriority=Low  PositionTargetValue=init_toe_joint_l  PositionTargetValueUnits=rad  VelocityTargetSpecify=off  VelocityTargetPriority=High  VelocityTargetValue=0  VelocityTargetValueUnits=deg/s
  Revolute2 : sm_lib/Joints/Revolute Joint  SenseConstraintForce=off  SenseConstraintForceX=off  SenseConstraintForceY=off  SenseConstraintForceZ=off  SenseConstraintTorque=off  SenseConstraintTorqueX=off  SenseConstraintTorqueY=off  SenseConstraintTorqueZ=off  SenseTotalForce=on  SenseTotalForceX=off  SenseTotalForceY=off  SenseTotalForceZ=off  SenseTotalTorque=off  SenseTotalTorqueX=off  SenseTotalTorqueY=off  SenseTotalTorqueZ=off  CompositeWrenchDir=FollowerOnBase  CompositeWrenchFrame=BaseFrame  EquilibriumPosition=0  EquilibriumPositionUnits=rad  SpringStiffness=0  SpringStiffnessUnits=m*N/rad  DampingCoefficient=0  DampingCoefficientUnits=m*s*N/rad  TorqueActuationMode=InputTorque  MotionActuationMode=ComputedMotion  SensePosition=off  SenseVelocity=on  SenseAcceleration=off  SenseTorqueForce=off  PositionTargetSpecify=off  PositionTargetPriority=Low  PositionTargetValue=minitaurParams.RevoluteJoint(3).Rz.Pos  PositionTargetValueUnits=deg  VelocityTargetSpecify=off  VelocityTargetPriority=High  VelocityTargetValue=0  VelocityTargetValueUnits=deg/s
  Revolute3 : sm_lib/Joints/Revolute Joint  SenseConstraintForce=off  SenseConstraintForceX=off  SenseConstraintForceY=off  SenseConstraintForceZ=off  SenseConstraintTorque=off  SenseConstraintTorqueX=off  SenseConstraintTorqueY=off  SenseConstraintTorqueZ=off  SenseTotalForce=on  SenseTotalForceX=off  SenseTotalForceY=off  SenseTotalForceZ=off  SenseTotalTorque=off  SenseTotalTorqueX=off  SenseTotalTorqueY=off  SenseTotalTorqueZ=off  CompositeWrenchDir=FollowerOnBase  CompositeWrenchFrame=BaseFrame  EquilibriumPosition=0  EquilibriumPositionUnits=rad  SpringStiffness=0  SpringStiffnessUnits=m*N/rad  DampingCoefficient=0  DampingCoefficientUnits=m*s*N/rad  TorqueActuationMode=InputTorque  MotionActuationMode=ComputedMotion  SensePosition=off  SenseVelocity=on  SenseAcceleration=off  SenseTorqueForce=off  PositionTargetSpecify=off  PositionTargetPriority=Low  PositionTargetValue=minitaurParams.RevoluteJoint(3).Rz.Pos  PositionTargetValueUnits=deg  VelocityTargetSpecify=off  VelocityTargetPriority=High  VelocityTargetValue=0  VelocityTargetValueUnits=deg/s
  Transform : sm_lib/Frames and Transforms/Rigid Transform  TranslationMethod=Cartesian  TranslationLengthUnit=mm  TranslationStandardAxis=+Z  TranslationStandardOffset=0  TranslationCartesianOffset=minitaurParams.RigidTransform(16).translation  TranslationROffset=0  TranslationROffsetUnits=m  TranslationZOffset=0  TranslationZOffsetUnits=m  TranslationThetaOffset=0  TranslationThetaOffsetUnits=deg  RotationMethod=ArbitraryAxis  RotationAngleUnits=rad  RotationStandardAxis=+Z  RotationAngle=minitaurParams.RigidTransform(16).angle  RotationArbitraryAxis=minitaurParams.RigidTransform(16).axis  FollAlignAxisA=+X  BaseAlignAxisA=+Y  FollAlignAxisB=+Y  BaseAlignAxisB=+Z  RotationSequenceAxes=FollowerAxes  RotationSequence=XYX  RotationSequenceAngles=[0 0 0]  RotationSequenceAnglesUnits=deg  RotationMatrix=[1 0 0; 0 1 0; 0 0 1]
  minitaur_leg_joint_placeholder_sim_1_RIGID : Subsystem
  minitaur_leg_joint_placeholder_sim_2_RIGID : Subsystem
  minitaur_leg_joint_placeholder_sim_3_RIGID : Subsystem
  minitaur_leg_lower_link_1_RIGID : Subsystem
  minitaur_leg_lower_link_toe_1_RIGID : Subsystem
  minitaur_leg_upper_link_2_RIGID : Subsystem
  minitaur_leg_upper_link_3_RIGID : Subsystem
  x2517T32_2_RIGID : Subsystem
  F1 : PMIOPort  Port=1  Side=Left
  F : PMIOPort  Port=2  Side=Left
  F_contact : PMIOPort  Port=3  Side=Right
  connections:
  minitaur_leg_upper_link_3_RIGID/RConn1 -- Revolute3/LConn1
  ReferenceFrame/RConn1 -- Transform/LConn1
  Transform/RConn1 -- minitaur_leg_upper_link_2_RIGID/LConn1
  minitaur_leg_upper_link_2_RIGID/LConn2 -- F/RConn1
  minitaur_leg_upper_link_3_RIGID/LConn1 -- F1/RConn1
  Revolute1/LConn1 -- minitaur_leg_lower_link_toe_1_RIGID/RConn2
  minitaur_leg_joint_placeholder_sim_2_RIGID/LConn1 -- minitaur_leg_lower_link_toe_1_RIGID/LConn2
  Revolute2/LConn1 -- minitaur_leg_lower_link_toe_1_RIGID/RConn1
  x2517T32_2_RIGID/LConn1 -- minitaur_leg_lower_link_toe_1_RIGID/LConn1
  minitaur_leg_joint_placeholder_sim_1_RIGID/LConn1 -- minitaur_leg_upper_link_3_RIGID/LConn2
  minitaur_leg_joint_placeholder_sim_3_RIGID/LConn1 -- minitaur_leg_upper_link_2_RIGID/LConn4
  F_contact/RConn1 -- x2517T32_2_RIGID/RConn1
  Revolute1/RConn1 -- minitaur_leg_lower_link_1_RIGID/LConn1
  Revolute2/RConn1 -- minitaur_leg_upper_link_2_RIGID/LConn3
  minitaur_leg_lower_link_1_RIGID/LConn2 -- Revolute3/RConn1
  Revolute2/LConn2 -- Joint Friction Model/RConn1
  Joint Friction Model2/LConn2 -- Revolute3/RConn3
  Revolute1/RConn2 -- Joint Friction Model1/LConn1
  Joint Friction Model2/LConn1 -- Revolute3/RConn2
  Revolute1/RConn3 -- Joint Friction Model1/LConn2
  Revolute1/LConn2 -- Joint Friction Model1/RConn1
  Joint Friction Model2/RConn1 -- Revolute3/LConn2
  Revolute2/RConn2 -- Joint Friction Model/LConn1
  Revolute2/RConn3 -- Joint Friction Model/LConn2
